simulink library "WZM_QSS_Lib"  (Simulink 7.7)
settings: Solver=ode45  StartTime=0.0  StopTime=10.0  RelTol=1e-3
undefined symbols (not defined in the file): A, AirCompressor, CNC, Housing, HydraulicPump, MainDrive, MainDriveCoolingEx, Process, ProcessCooling, R
libraries: WZM_QSS_Lib x36
(part 2 of 2)

== system WZM_QSS_Lib/ThermalManagement/MainDriveCoolingEx/Temperatur ==
  Q_Spindel : Inport
  Q_Kuehlung : Inport  Port=2
  Theta_amb [K] : Inport  Port=3
  Add : Sum  Inputs=+--
  Gain : Gain  Gain=1/m/cp
  Gain1 : Gain  Gain=R*A
  Integrator Limited : Integrator  InitialConditionSource=external  LimitOutput=on
  Sum : Sum  Inputs=|-+
  T [K] : Outport
  Qdot_Oberflaeche [W] : Outport  Port=2
  wires:
  Q_Kuehlung/1 -> Add/2
  Theta_amb [K]/1 -> Integrator Limited/2, Sum/1
  Q_Spindel/1 -> Add/1
  Gain1/1 -> Qdot_Oberflaeche [W]/1, Add/3
  Sum/1 -> Gain1/1
  Integrator Limited/1 -> Sum/2, T [K]/1
  Gain/1 -> Integrator Limited/1
  Add/1 -> Gain/1
